simulink model "dyn2"  (R2021b)
settings: Solver=VariableStepAuto  StartTime=0.0  StopTime=10.0  RelTol=1e-3
InitFcn:
  | m=5;
  | I=[0.5 0 0; 0 0.5 0; 0 0 1];
  | c_t=0.02;
  | c_m=0.005;
  | h_i=10;
  | g=9.80665;
  | rho=1;
  | omega_hover=sqrt(m*g/(4*0.5*c_t));
  | a_x=0;
  | a_y=0;
  | a_z=0;
  | a_r=0;
  | a_p=0;
  | a_yaw=0;
  | casee=1;
  | x_i=0;
  | y_i=0;
  | z_i=-10;
  | r_i=0;
  | p_i=90;
  | yaw_i=0;
  | x_f=1;
  | y_f=0;
  | z_f=-10;
  | r_f=0;
  | p_f=90;
  | yaw_f=0;
undefined symbols (not defined in the file or in its folder): X, Y, Z
libraries: sm_lib x32, nesl_utility x11, slpidlib x6
(part 1 of 2)
settings Model: Creator=zafar  LastModifiedBy=zafar

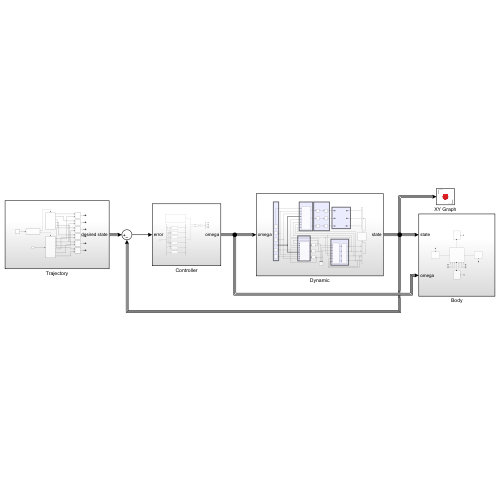
[thumbnail: Simulink's stored preview of the top-level diagram]
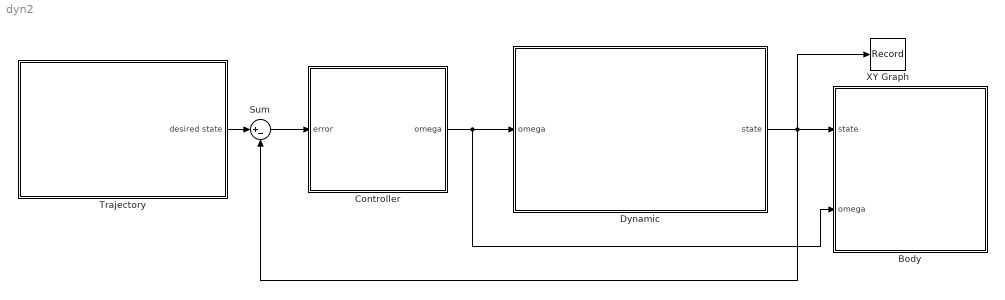
== system dyn2 ==
  Body : Subsystem
  Controller : Subsystem
  Dynamic : Subsystem
  Sum : Sum  Inputs=|+-
  Trajectory : Subsystem
  XY Graph : Record  FileSettingsInternal="{\"entries\":[{\"content\":{\"excelSettings\":{\"content\":{},\"type\":\"Streamout.ExcelSettings\"}},\"type\":\"Streamout.FileSettingStorage\",\"uuid\":\"d4792fb1-0a1f-4ec5-b838-d1a9abcf2949\"}],\"packageUris\":[\"http://schema.mathworks.com/mf0/streamout_blocks/R2020a\"],\"version\":\"1.0\"}"  Layout=[1 2]  SignalsInternal="{\"entries\":[{\"content\":{\"signals\":[{\"content\":{\"blockPath\":[\"dyn2/XY Graph\"],\"channel\":[],\"dimensions\":[1],\"domain\":\"dyn2/XY Graph\",\"hasChildren\":true,\"lineColor\":\"#139fff\",\"plots\":[],\"port\":1,\"sid\":[\"\"],\"signalID\":683,\"signalName\":\"Dynamic\"},\"type\":\"RecordBlkView.Signal\",\"uuid\":\"e1957810-dc31-4c74-8302-1d5d707b7b59\"},{\"content\":{\"blockPath\":[\"dyn2/XY Graph\"],\"channel\":[],\"dimensions\":[1],\"domain\":\"dyn2/XY Graph\",\"leafPath\":\"Dynamic.roll\",\"lineColor\":\"#ff6929\",\"parentID\":683,\"plots\":[9],\"port\":1,\"sid\":[\"\"],\"signalID\":689,\"signalName\":\"Dynamic.roll\"},\"type\":\"RecordBlkView.Signal\",\"uuid\":\"85618280-ea2e-4b5a-aaad-2ba74497e0b1\"},{\"content\":{\"blockPath\":[\"dyn2/XY Graph\"],\"channel\":[],\"dimensions\":[1],\"domain\":\"dyn2/XY Graph\",\"leafPath\":\"Dynamic.pitch\",\"lineColor\":\"#b746ff\",\"parentID\":683,\"plots\":[9],\"port\":1,\"sid\":[\"\"],\"signalID\":693,\"signalName\":\"Dynamic.pitch\"},\"type\":\"RecordBlkView.Signal\",\"uuid\":\"18941b2a-ec3b-4b33-bc23-00b06118022f\"},{\"content\":{\"blockPath\":[\"dyn2/XY Graph\"],\"channel\":[],\"dimensions\":[1],\"domain\":\"dyn2/XY Graph\",\"leafPath\":\"Dynamic.yaw\",\"lineColor\":\"#64d413\",\"parentID\":683,\"plots\":[9],\"port\":1,\"sid\":[\"\"],\"signalID\":697,\"signalName\":\"Dynamic.yaw\"},\"type\":\"RecordBlkView.Signal\",\"uuid\":\"7d2db7da-f018-4d39-9722-8c8cb8260ba4\"},{\"content\":{\"blockPath\":[\"dyn2/XY Graph\"],\"channel\":[],\"dimensions\":[1],\"domain\":\"dyn2/XY Graph\",\"leafPath\":\"Dynamic.x\",\"lineColor\":\"#ff13a6\",\"parentID\":683,\"plots\":[1],\"port\":1,\"sid\":[\"\"],\"signalID\":701,\"signalName\":\"Dynamic.x\"},\"type\":\"RecordBlkView.Signal\",\"uuid\":\"06cf0755-9d67-498c-9d15-2dd6aaf754d1\"},{\"content\":{\"blockPath\":[\"dyn2/XY Graph\"],\"channel\":[],\"dimensions\":[1],\"domain\":\"dyn2/XY Graph\",\"leafPath\":\"Dynamic.y\",\"lineColor\":\"#fe330a\",\"parentID\":683,\"plots\":[1],\"port\":1,\"sid\":[\"\"],\"signalID\":705,\"signalName\":\"Dynamic.y\"},\"type\":\"RecordBlkView.Signal\",\"uuid\":\"010e3232-da4b-4a82-8d08-832df45afe02\"},{\"content\":{\"blockPath\":[\"dyn2/XY Graph\"],\"channel\":[],\"dimensions\":[1],\"domain\":\"dyn2/XY Graph\",\"leafPath\":\"Dynamic.z\",\"lineColor\":\"#22b573\",\"parentID\":683,\"plots\":[1],\"port\":1,\"sid\":[\"\"],\"signalID\":709,\"signalName\":\"Dynamic.z\"},\"type\":\"RecordBlkView.Signal\",\"uuid\":\"f4e3abf7-5929-44e1-b69c-6cdf4737284f\"}]},\"type\":\"RecordBlkView.InputSignals\",\"uuid\":\"78fd29e7-ed61-4860-890e-9c6bc17d912c\"}],\"packageUris\":[\"http://schema.mathworks.com/mf0/streamout_blocks/R2020a\"],\"version\":\"1.0\"}"  CompatibilityTag=XY
  wires:
  Dynamic/1(state) -> XY Graph/1, Sum/2, Body/1(state)
  Controller/1(omega) -> Body/2(omega), Dynamic/1(omega)
  Trajectory/1(desired state) -> Sum/1
  Sum/1 -> Controller/1(error)

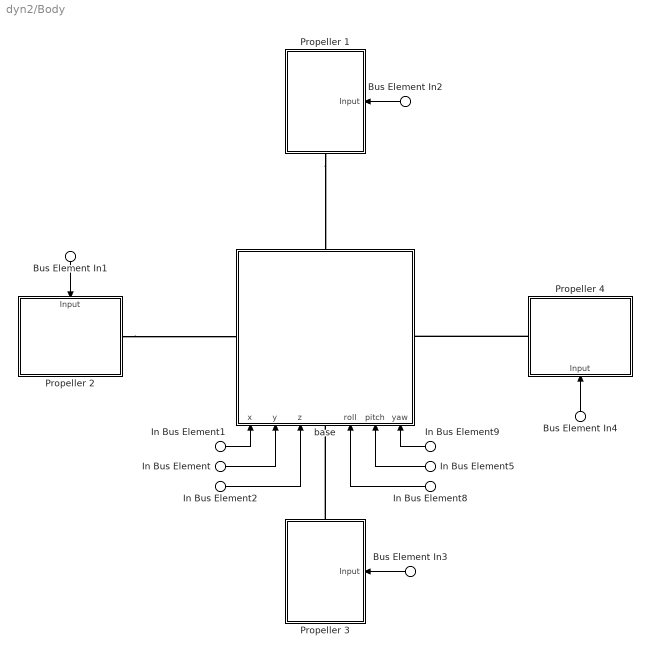
== system dyn2/Body ==
  In Bus Element2 : Inport  PortName=state  Element=z
  In Bus Element1 : Inport  PortName=state  Element=x
  In Bus Element9 : Inport  PortName=state  Element=yaw
  In Bus Element8 : Inport  PortName=state  Element=roll
  In Bus Element5 : Inport  PortName=state  Element=pitch
  In Bus Element : Inport  PortName=state  Element=y
  Bus Element In2 : Inport  Port=2  PortName=omega  Element=omega1
  Bus Element In1 : Inport  Port=2  PortName=omega  Element=omega2
  Bus Element In3 : Inport  Port=2  PortName=omega  Element=omega3
  Bus Element In4 : Inport  Port=2  PortName=omega  Element=omega4
  Propeller 1 : Subsystem
      settings: PortSchema="{\"entries\":[{\"content\":{\"sides\":[{\"content\":{\"connectorIds\":[\"LConn1\"]},\"type\":\"ConnectorPlacement.EquallySpacedRectSide\",\"uuid\":\"cdf25c99-c2c9-48d7-87ea-f6e3a99d1ccc\"},{\"content\":{\"connectorIds\":[],\"side\":\"RIGHT\"},\"type\":\"ConnectorPlacement.EquallySpacedRectSide\",\"uuid\":\"40e1c002-c04a-4a5a-8e9c-b357988226a7\"},{\"content\":{\"connectorIds\":[],\"side\":\"TOP\"},\"type\":\"ConnectorPlacement.EquallySpacedRectSide\",\"uuid\":\"eab61d94-1bf1-42a1-b49f-e701cda87405\"},{\"content\":{\"connectorIds\":[\"In1\"],\"side\":\"BOTTOM\"},\"type\":\"ConnectorPlacement.EquallySpacedRectSide\",\"uuid\":\"d4baf7fe-500e-43b3-b49d-f7ceb4534939\"}]},\"type\":\"ConnectorPlacement.EquallySpacedConnector\",\"uuid\":\"1942d34c-f553-4d78-8efb-5354772d0834\"}],\"packageUris\":[\"http://schema.mathworks.com/mf0/Connector/R2020b\"],\"version\":\"1.0\"}"
  Propeller 2 : Subsystem
      settings: PortSchema="{\"entries\":[{\"content\":{\"sides\":[{\"content\":{\"connectorIds\":[\"LConn1\"]},\"type\":\"ConnectorPlacement.EquallySpacedRectSide\",\"uuid\":\"cdf25c99-c2c9-48d7-87ea-f6e3a99d1ccc\"},{\"content\":{\"connectorIds\":[],\"side\":\"RIGHT\"},\"type\":\"ConnectorPlacement.EquallySpacedRectSide\",\"uuid\":\"40e1c002-c04a-4a5a-8e9c-b357988226a7\"},{\"content\":{\"connectorIds\":[\"In1\"],\"side\":\"TOP\"},\"type\":\"ConnectorPlacement.EquallySpacedRectSide\",\"uuid\":\"eab61d94-1bf1-42a1-b49f-e701cda87405\"}]},\"type\":\"ConnectorPlacement.EquallySpacedConnector\",\"uuid\":\"1942d34c-f553-4d78-8efb-5354772d0834\"}],\"packageUris\":[\"http://schema.mathworks.com/mf0/Connector/R2020b\"],\"version\":\"1.0\"}"
  Propeller 3 : Subsystem
      settings: PortSchema="{\"entries\":[{\"content\":{\"sides\":[{\"content\":{\"connectorIds\":[\"LConn1\"]},\"type\":\"ConnectorPlacement.EquallySpacedRectSide\",\"uuid\":\"cdf25c99-c2c9-48d7-87ea-f6e3a99d1ccc\"},{\"content\":{\"connectorIds\":[],\"side\":\"RIGHT\"},\"type\":\"ConnectorPlacement.EquallySpacedRectSide\",\"uuid\":\"40e1c002-c04a-4a5a-8e9c-b357988226a7\"},{\"content\":{\"connectorIds\":[],\"side\":\"TOP\"},\"type\":\"ConnectorPlacement.EquallySpacedRectSide\",\"uuid\":\"eab61d94-1bf1-42a1-b49f-e701cda87405\"},{\"content\":{\"connectorIds\":[\"In1\"],\"side\":\"BOTTOM\"},\"type\":\"ConnectorPlacement.EquallySpacedRectSide\",\"uuid\":\"d7470312-54f3-4d3a-8a81-0efcc21151e7\"}]},\"type\":\"ConnectorPlacement.EquallySpacedConnector\",\"uuid\":\"1942d34c-f553-4d78-8efb-5354772d0834\"}],\"packageUris\":[\"http://schema.mathworks.com/mf0/Connector/R2020b\"],\"version\":\"1.0\"}"
  Propeller 4 : Subsystem
      settings: PortSchema="{\"entries\":[{\"content\":{\"sides\":[{\"content\":{\"connectorIds\":[\"LConn1\"]},\"type\":\"ConnectorPlacement.EquallySpacedRectSide\",\"uuid\":\"cdf25c99-c2c9-48d7-87ea-f6e3a99d1ccc\"},{\"content\":{\"connectorIds\":[],\"side\":\"RIGHT\"},\"type\":\"ConnectorPlacement.EquallySpacedRectSide\",\"uuid\":\"40e1c002-c04a-4a5a-8e9c-b357988226a7\"},{\"content\":{\"connectorIds\":[],\"side\":\"TOP\"},\"type\":\"ConnectorPlacement.EquallySpacedRectSide\",\"uuid\":\"eab61d94-1bf1-42a1-b49f-e701cda87405\"},{\"content\":{\"connectorIds\":[\"In1\"],\"side\":\"BOTTOM\"},\"type\":\"ConnectorPlacement.EquallySpacedRectSide\",\"uuid\":\"25618f8e-b249-4005-b2d0-d585f13f3048\"}]},\"type\":\"ConnectorPlacement.EquallySpacedConnector\",\"uuid\":\"1942d34c-f553-4d78-8efb-5354772d0834\"}],\"packageUris\":[\"http://schema.mathworks.com/mf0/Connector/R2020b\"],\"version\":\"1.0\"}"
  base : Subsystem
      settings: PortSchema="{\"entries\":[{\"content\":{\"sides\":[{\"content\":{\"connectorIds\":[\"In1\",\"In2\",\"In3\",\"LConn1\",\"In4\",\"In5\",\"In6\"]},\"type\":\"ConnectorPlacement.EquallySpacedRectSide\",\"uuid\":\"779db686-b372-48f2-8e56-3039c1dfa828\"},{\"content\":{\"connectorIds\":[\"RConn1\"],\"side\":\"RIGHT\"},\"type\":\"ConnectorPlacement.EquallySpacedRectSide\",\"uuid\":\"5342d4b0-d4cc-41da-a1a0-0c3712086a6a\"},{\"content\":{\"connectorIds\":[\"LConn2\"],\"side\":\"TOP\"},\"type\":\"ConnectorPlacement.EquallySpacedRectSide\",\"uuid\":\"806fe2cc-07c0-46bb-9d80-26a95cc2c32b\"},{\"content\":{\"connectorIds\":[\"RConn2\"],\"side\":\"BOTTOM\"},\"type\":\"ConnectorPlacement.EquallySpacedRectSide\",\"uuid\":\"aa12e65d-c8a8-4fde-8e0f-187926b8e052\"}]},\"type\":\"ConnectorPlacement.EquallySpacedConnector\",\"uuid\":\"4d2b6a53-689c-48c9-b350-3dab09cbcb7b\"}],\"packageUris\":[\"http://schema.mathworks.com/mf0/Connector/R2020b\"],\"version\":\"1.0\"}"
  wires:
  In Bus Element1/1 -> base/1(x)
  In Bus Element/1 -> base/2(y)
  In Bus Element2/1 -> base/3(z)
  In Bus Element8/1 -> base/4(roll)
  In Bus Element5/1 -> base/5(pitch)
  In Bus Element9/1 -> base/6(yaw)
  Bus Element In2/1 -> Propeller 1/1(Input)
  Bus Element In1/1 -> Propeller 2/1(Input)
  Bus Element In3/1 -> Propeller 3/1(Input)
  Bus Element In4/1 -> Propeller 4/1(Input)
  connections:
  Propeller 4/LConn1 -- base/RConn2
  Propeller 1/LConn1 -- base/RConn1
  Propeller 2/LConn1 -- base/LConn2
  Propeller 3/LConn1 -- base/LConn1

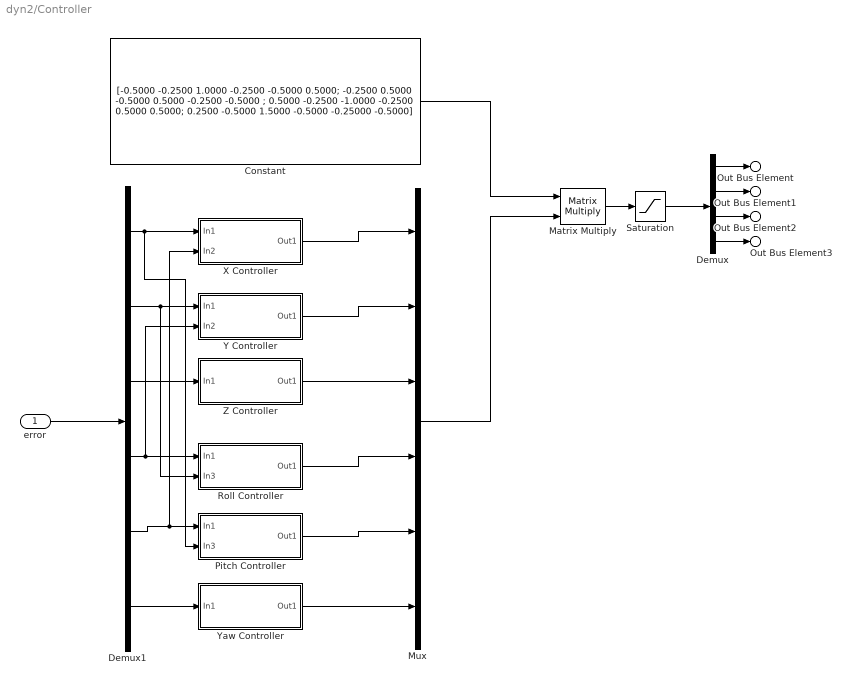
== system dyn2/Controller ==
  error : Inport
  Constant : Constant  Value=|
      | [-0.5000   -0.2500    1.0000   -0.2500   -0.5000    0.5000;
      |    -0.2500    0.5000   -0.5000    0.5000   -0.2500   -0.5000
      | ;    0.5000   -0.2500   -1.0000   -0.2500    0.5000    0.5000;
      |     0.2500   -0.5000    1.5000   -0.5000   -0.25000   -0.5000]
  Demux : Demux
  Demux1 : Demux  Outputs=6
  Matrix Multiply : Product  Multiplication=Matrix(*)
  Mux : Mux  Inputs=6
  Pitch Controller : Subsystem
  Roll Controller : Subsystem
  Saturation : Saturate  UpperLimit=10000  LowerLimit=0
  X Controller : Subsystem
  Y Controller : Subsystem
  Yaw Controller : Subsystem
  Z Controller : Subsystem
  Out Bus Element : Outport  PortName=omega  Element=omega1
  Out Bus Element1 : Outport  PortName=omega  Element=omega2
  Out Bus Element2 : Outport  PortName=omega  Element=omega3
  Out Bus Element3 : Outport  PortName=omega  Element=omega4
  wires:
  Yaw Controller/1(Out1) -> Mux/6
  Pitch Controller/1(Out1) -> Mux/5
  Roll Controller/1(Out1) -> Mux/4
  Z Controller/1(Out1) -> Mux/3
  X Controller/1(Out1) -> Mux/1
  Constant/1 -> Matrix Multiply/1
  Mux/1 -> Matrix Multiply/2
  Matrix Multiply/1 -> Saturation/1
  Saturation/1 -> Demux/1
  Demux/1 -> Out Bus Element/1
  Demux/2 -> Out Bus Element1/1
  Demux/3 -> Out Bus Element2/1
  Demux/4 -> Out Bus Element3/1
  Demux1/1 -> Pitch Controller/2(In3), X Controller/1(In1)
  Demux1/3 -> Z Controller/1(In1)
  Demux1/4 -> Y Controller/2(In2), Roll Controller/1(In1)
  Demux1/5 -> X Controller/2(In2), Pitch Controller/1(In1)
  Demux1/6 -> Yaw Controller/1(In1)
  error/1 -> Demux1/1
  Demux1/2 -> Roll Controller/2(In3), Y Controller/1(In1)
  Y Controller/1(Out1) -> Mux/2

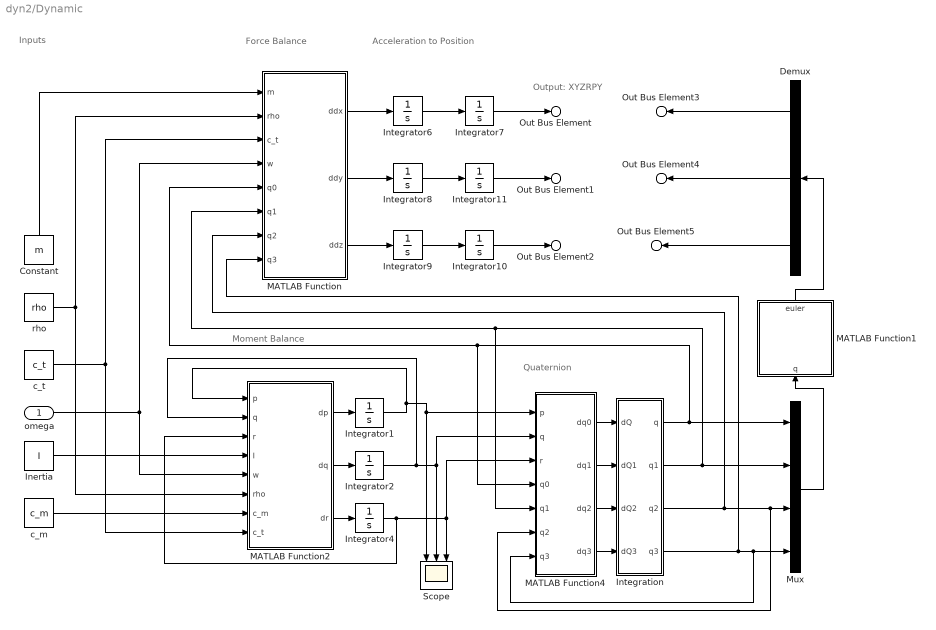
== system dyn2/Dynamic ==
  note: Inputs
  note: Moment Balance
  note: Quaternion
  note: Acceleration to Position
  note: Force Balance
  note: Output: XYZRPY
  omega : Inport
  Constant : Constant  Value=m
  Demux : Demux  Outputs=3
  Inertia : Constant  Value=I
  Integration : Subsystem
  Integrator{1..2,4,6..9,11} (8 alike) : Integrator
  Integrator10 : Integrator  InitialCondition=-h_i
  MATLAB Function : MATLAB Function  TreatAsAtomicUnit=on
  MATLAB Function1 : MATLAB Function  TreatAsAtomicUnit=on
  MATLAB Function2 : MATLAB Function  TreatAsAtomicUnit=on
  MATLAB Function4 : MATLAB Function  TreatAsAtomicUnit=on
  Mux : Mux
  Scope : Scope  NumInputPorts=3
  c_m : Constant  Value=c_m
  c_t : Constant  Value=c_t
  rho : Constant  Value=rho
  Out Bus Element3 : Outport  PortName=state  Element=roll
  Out Bus Element4 : Outport  PortName=state  Element=pitch
  Out Bus Element5 : Outport  PortName=state  Element=yaw
  Out Bus Element : Outport  PortName=state  Element=x
  Out Bus Element1 : Outport  PortName=state  Element=y
  Out Bus Element2 : Outport  PortName=state  Element=z
  wires:
  Mux/1 -> MATLAB Function1/1(q)
  Integration/4(q3) -> Mux/4, MATLAB Function4/7(q3), MATLAB Function/8(q3)
  Integration/3(q2) -> Mux/3, MATLAB Function4/6(q2), MATLAB Function/7(q2)
  Integration/2(q1) -> Mux/2, MATLAB Function4/5(q1), MATLAB Function/6(q1)
  MATLAB Function4/4(dq3) -> Integration/4(dQ3)
  MATLAB Function4/3(dq2) -> Integration/3(dQ2)
  MATLAB Function4/2(dq1) -> Integration/2(dQ1)
  MATLAB Function4/1(dq0) -> Integration/1(dQ)
  Demux/2 -> Out Bus Element4/1
  Demux/3 -> Out Bus Element5/1
  Integrator4/1 -> MATLAB Function4/3(r), Scope/3, MATLAB Function2/3(r)
  MATLAB Function1/1(euler) -> Demux/1
  MATLAB Function/2(ddy) -> Integrator8/1
  Demux/1 -> Out Bus Element3/1
  Constant/1 -> MATLAB Function/1(m)
  rho/1 -> MATLAB Function2/6(rho), MATLAB Function/2(rho)
  c_m/1 -> MATLAB Function2/7(c_m)
  MATLAB Function/3(ddz) -> Integrator9/1
  Integrator1/1 -> MATLAB Function4/1(p), Scope/1, MATLAB Function2/1(p)
  Integration/1(q) -> Mux/1, MATLAB Function4/4(q0), MATLAB Function/5(q0)
  MATLAB Function2/1(dp) -> Integrator1/1
  Integrator10/1 -> Out Bus Element2/1
  MATLAB Function/1(ddx) -> Integrator6/1
  Integrator8/1 -> Integrator11/1
  MATLAB Function2/2(dq) -> Integrator2/1
  Integrator6/1 -> Integrator7/1
  Integrator11/1 -> Out Bus Element1/1
  Integrator7/1 -> Out Bus Element/1
  Integrator2/1 -> MATLAB Function2/2(q), Scope/2, MATLAB Function4/2(q)
  c_t/1 -> MATLAB Function2/8(c_t), MATLAB Function/3(c_t)
  Integrator9/1 -> Integrator10/1
  omega/1 -> MATLAB Function/4(w), MATLAB Function2/5(w)
  MATLAB Function2/3(dr) -> Integrator4/1
  Inertia/1 -> MATLAB Function2/4(I)

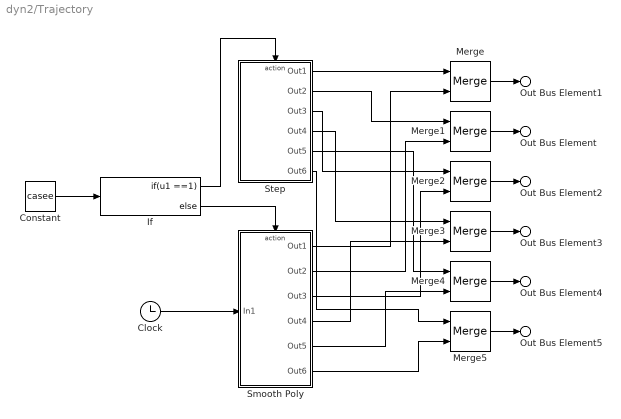
== system dyn2/Trajectory ==
  Clock : Clock
  Constant : Constant  Value=casee
  If : If  IfExpression=u1 ==1
  Merge{,1..5} (6 alike) : Merge
  Smooth Poly : Subsystem  TreatAsAtomicUnit=on
  Step : Subsystem  TreatAsAtomicUnit=on
  Out Bus Element1 : Outport  PortName=desired state  Element=x
  Out Bus Element : Outport  PortName=desired state  Element=y
  Out Bus Element2 : Outport  PortName=desired state  Element=z
  Out Bus Element3 : Outport  PortName=desired state  Element=roll
  Out Bus Element4 : Outport  PortName=desired state  Element=pitch
  Out Bus Element5 : Outport  PortName=desired state  Element=yaw
  wires:
  Smooth Poly/3(Out3) -> Merge2/2
  Step/3(Out3) -> Merge2/1
  Smooth Poly/2(Out2) -> Merge1/2
  Step/2(Out2) -> Merge1/1
  Smooth Poly/1(Out1) -> Merge/2
  Step/1(Out1) -> Merge/1
  If/2 -> Smooth Poly/Action
  If/1 -> Step/Action
  Constant/1 -> If/1
  Clock/1 -> Smooth Poly/1(In1)
  Step/4(Out4) -> Merge3/1
  Smooth Poly/4(Out4) -> Merge3/2
  Smooth Poly/5(Out5) -> Merge4/2
  Step/5(Out5) -> Merge4/1
  Step/6(Out6) -> Merge5/1
  Smooth Poly/6(Out6) -> Merge5/2
  Merge/1 -> Out Bus Element1/1
  Merge1/1 -> Out Bus Element/1
  Merge2/1 -> Out Bus Element2/1
  Merge3/1 -> Out Bus Element3/1
  Merge4/1 -> Out Bus Element4/1
  Merge5/1 -> Out Bus Element5/1

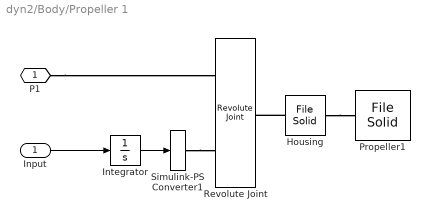
== system dyn2/Body/Propeller 1 ==
  Input : Inport
  Housing : sm_lib/Body Elements/File Solid  ExtGeomFileName=E:\tosort\aerial\my new version\motor.STEP  UnitType=FromFile  ExtGeomFileUnits=m  StepReaderType=HEX  ExportConvexHullGeometry=off  InertiaType=Custom  Mass=51  MassUnits=g  CenterOfMass=[0, 0, -0.0088876]  CenterOfMassUnits=m  MomentsOfInertia=[7.0438e-06, 7.04379e-06, 6.06908e-06]  MomentsOfInertiaUnits=kg*m^2  ProductsOfInertia=[0 0 0]  ProductsOfInertiaUnits=kg*m^2  BasedOnType=Mass  Density=1000  DensityUnits=kg/m^3  DoExposeReferenceFrame=off  SerializedFrames=<Frames><Frame><Id>Frame1</Id><Value><Name>F1</Name><Origin><Source>GeometricFeature</Source><FeatureName>planar surface 3</FeatureName></Origin><PrimaryAxis><DefinedDirection>+Z</DefinedDirection><Source>ReferenceFrame</Source><SourceDirection>+Z</SourceDirection><FeatureName></FeatureName></PrimaryAxis><SecondaryAxis><DefinedDirection>+X</DefinedDirection><Source>ReferenceFrame</Source><SourceDirection>+X</SourceDirection><FeatureName></FeatureName></SecondaryAxis></Value></Frame><Frame><Id>Frame2</Id><Value><Name>F2</Name><Origin><Source>GeometricFeature</Source><FeatureName>circular curve 1</FeatureName></Origin><PrimaryAxis><DefinedDirection>+Z</DefinedDirection><Source>ReferenceFrame</Source><SourceDirection>+Z</SourceDirection><FeatureName></FeatureName></PrimaryAxis><SecondaryAxis><DefinedDirection>+X</DefinedDirection><Source>ReferenceFrame</Source><SourceDirection>+X</SourceDirection><FeatureName></FeatureName></SecondaryAxis></Value></Frame></Frames>  GraphicType=FromGeometry  MarkerShape=Sphere  MarkerSize=10  GraphicVisPropType=SimpleVisualProperties  GraphicDiffuseColor=[0.6 0.0 0.2]  GraphicSpecularColor=[0.5 0.5 0.5 1.0]  GraphicAmbientColor=[0.15 0.15 0.15 1.0]  GraphicEmissiveColor=[0.0 0.0 0.0 1.0]  GraphicShininess=75  GraphicOpacity=1.0
  Integrator : Integrator
  Propeller1 : sm_lib/Body Elements/File Solid  ExtGeomFileName=E:\tosort\aerial\my new version\propeller.STEP  UnitType=FromFile  ExtGeomFileUnits=m  StepReaderType=HEX  ExportConvexHullGeometry=off  InertiaType=Custom  Mass=0.0249468  MassUnits=kg  CenterOfMass="[0  0.00566766 0]"  CenterOfMassUnits=m  MomentsOfInertia=[0.000160013, 0.000160582, 8.20018e-07]  MomentsOfInertiaUnits=kg*m^2  ProductsOfInertia=[0 0 0]  ProductsOfInertiaUnits=kg*m^2  BasedOnType=Density  Density=1  DensityUnits=g/cm^3  DoExposeReferenceFrame=off  SerializedFrames=<Frames><Frame><Id>Frame1</Id><Value><Name>F1</Name><Origin><Source>GeometricFeature</Source><FeatureName>circular curve 14</FeatureName></Origin><PrimaryAxis><DefinedDirection>+Z</DefinedDirection><Source>ReferenceFrame</Source><SourceDirection>+Y</SourceDirection><FeatureName></FeatureName></PrimaryAxis><SecondaryAxis><DefinedDirection>+X</DefinedDirection><Source>ReferenceFrame</Source><SourceDirection>+X</SourceDirection><FeatureName></FeatureName></SecondaryAxis></Value></Frame></Frames>  GraphicType=FromGeometry  MarkerShape=Sphere  MarkerSize=10  GraphicVisPropType=AdvancedVisualProperties  GraphicDiffuseColor=[0.05 0.05 0.05]  GraphicSpecularColor=[0.5 0.5 0.5 1.0]  GraphicAmbientColor=[0.15 0.15 0.15 1.0]  GraphicEmissiveColor=[0.0 0.0 0.0 1.0]  GraphicShininess=40  GraphicOpacity=1.0
  Revolute Joint : sm_lib/Joints/Revolute Joint  JointMode=Normal  SenseConstraintForce=off  SenseConstraintForceX=off  SenseConstraintForceY=off  SenseConstraintForceZ=off  SenseConstraintTorque=off  SenseConstraintTorqueX=off  SenseConstraintTorqueY=off  SenseConstraintTorqueZ=off  SenseTotalForce=off  SenseTotalForceX=off  SenseTotalForceY=off  SenseTotalForceZ=off  SenseTotalTorque=off  SenseTotalTorqueX=off  SenseTotalTorqueY=off  SenseTotalTorqueZ=off  CompositeWrenchDir=FollowerOnBase  CompositeWrenchFrame=BaseFrame  EquilibriumPosition=0  EquilibriumPositionUnits=deg  SpringStiffness=0  SpringStiffnessUnits=N*m/rad  DampingCoefficient=1e-5  DampingCoefficientUnits=N*m/(rad/s)  TorqueActuationMode=ComputedTorque  MotionActuationMode=InputMotion  SensePosition=off  SenseVelocity=off  SenseAcceleration=off  SenseTorqueForce=off  SenseLowerLimitTorqueForce=off  SenseUpperLimitTorqueForce=off  LowerLimitSpecify=off  LowerLimitBound=-90  LowerLimitBoundUnits=deg  LowerLimitStiffness=1e4  LowerLimitStiffnessUnits=N*m/deg  LowerLimitDamping=10  LowerLimitDampingUnits=N*m/(deg/s)  LowerLimitTransitionRegionWidth=0.1  LowerLimitTransitionRegionWidthUnits=deg  UpperLimitSpecify=off  UpperLimitBound=90  UpperLimitBoundUnits=deg  UpperLimitStiffness=1e4  UpperLimitStiffnessUnits=N*m/deg  UpperLimitDamping=10  UpperLimitDampingUnits=N*m/(deg/s)  UpperLimitTransitionRegionWidth=0.1  UpperLimitTransitionRegionWidthUnits=deg  PositionTargetSpecify=off  PositionTargetPriority=High  PositionTargetValue=0  PositionTargetValueUnits=deg  VelocityTargetSpecify=off  VelocityTargetPriority=High  VelocityTargetValue=0  VelocityTargetValueUnits=deg/s
  Simulink-PS Converter1 : nesl_utility/Simulink-PS Converter  PhysicalDomain=network_engine_domain  SubClassName=ps_input  LeftPortType=input  RightPortType=output  PseudoPeriodic=off  Frequencies=[]  NoiseDistribution=none  NoiseParameters=[]  Unit=rad  AffineConversion=off  FilteringAndDerivatives=filter  SimscapeFilterOrder=2  InputFilterTimeConstant=0.001  UdotUserProvided=0
      settings: SourceProductBaseCode=PW,SS
  P1 : PMIOPort  Side=Left
  wires:
  Input/1 -> Integrator/1
  Integrator/1 -> Simulink-PS Converter1/1
  connections:
  Housing/RConn1 -- Propeller1/LConn1
  P1/RConn1 -- Revolute Joint/LConn1
  Housing/LConn1 -- Revolute Joint/RConn1
  Simulink-PS Converter1/RConn1 -- Revolute Joint/LConn2

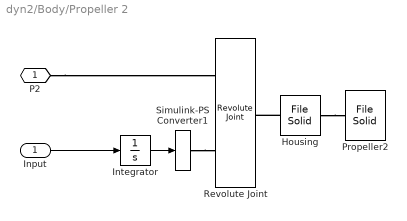
== system dyn2/Body/Propeller 2 ==
  Input : Inport
  Housing : sm_lib/Body Elements/File Solid  ExtGeomFileName=E:\tosort\aerial\my new version\motor.STEP  UnitType=FromFile  ExtGeomFileUnits=m  StepReaderType=HEX  ExportConvexHullGeometry=off  InertiaType=Custom  Mass=51  MassUnits=g  CenterOfMass=[0, 0, -0.0088876]  CenterOfMassUnits=m  MomentsOfInertia=[7.0438e-06, 7.04379e-06, 6.06908e-06]  MomentsOfInertiaUnits=kg*m^2  ProductsOfInertia=[0 0 0]  ProductsOfInertiaUnits=kg*m^2  BasedOnType=Mass  Density=1000  DensityUnits=kg/m^3  DoExposeReferenceFrame=off  SerializedFrames=<Frames><Frame><Id>Frame1</Id><Value><Name>F1</Name><Origin><Source>GeometricFeature</Source><FeatureName>planar surface 3</FeatureName></Origin><PrimaryAxis><DefinedDirection>+Z</DefinedDirection><Source>ReferenceFrame</Source><SourceDirection>+Z</SourceDirection><FeatureName></FeatureName></PrimaryAxis><SecondaryAxis><DefinedDirection>+X</DefinedDirection><Source>ReferenceFrame</Source><SourceDirection>+X</SourceDirection><FeatureName></FeatureName></SecondaryAxis></Value></Frame><Frame><Id>Frame2</Id><Value><Name>F2</Name><Origin><Source>GeometricFeature</Source><FeatureName>circular curve 1</FeatureName></Origin><PrimaryAxis><DefinedDirection>+Z</DefinedDirection><Source>ReferenceFrame</Source><SourceDirection>+Z</SourceDirection><FeatureName></FeatureName></PrimaryAxis><SecondaryAxis><DefinedDirection>+X</DefinedDirection><Source>ReferenceFrame</Source><SourceDirection>+X</SourceDirection><FeatureName></FeatureName></SecondaryAxis></Value></Frame></Frames>  GraphicType=FromGeometry  MarkerShape=Sphere  MarkerSize=10  GraphicVisPropType=SimpleVisualProperties  GraphicDiffuseColor=[0.6 0.0 0.2]  GraphicSpecularColor=[0.5 0.5 0.5 1.0]  GraphicAmbientColor=[0.15 0.15 0.15 1.0]  GraphicEmissiveColor=[0.0 0.0 0.0 1.0]  GraphicShininess=75  GraphicOpacity=1.0
  Integrator : Integrator
  Propeller2 : sm_lib/Body Elements/File Solid  ExtGeomFileName=E:\tosort\aerial\my new version\propeller.STEP  UnitType=FromFile  ExtGeomFileUnits=m  StepReaderType=HEX  ExportConvexHullGeometry=off  InertiaType=Custom  Mass=0.0249468  MassUnits=kg  CenterOfMass="[0  0.00566766 0]"  CenterOfMassUnits=m  MomentsOfInertia=[0.000160013, 0.000160582, 8.20018e-07]  MomentsOfInertiaUnits=kg*m^2  ProductsOfInertia=[0 0 0]  ProductsOfInertiaUnits=kg*m^2  BasedOnType=Density  Density=1  DensityUnits=g/cm^3  DoExposeReferenceFrame=off  SerializedFrames=<Frames><Frame><Id>Frame1</Id><Value><Name>F1</Name><Origin><Source>GeometricFeature</Source><FeatureName>circular curve 14</FeatureName></Origin><PrimaryAxis><DefinedDirection>+Z</DefinedDirection><Source>ReferenceFrame</Source><SourceDirection>+Y</SourceDirection><FeatureName></FeatureName></PrimaryAxis><SecondaryAxis><DefinedDirection>+X</DefinedDirection><Source>ReferenceFrame</Source><SourceDirection>+X</SourceDirection><FeatureName></FeatureName></SecondaryAxis></Value></Frame></Frames>  GraphicType=FromGeometry  MarkerShape=Sphere  MarkerSize=10  GraphicVisPropType=AdvancedVisualProperties  GraphicDiffuseColor=[0.05 0.05 0.05]  GraphicSpecularColor=[0.5 0.5 0.5 1.0]  GraphicAmbientColor=[0.15 0.15 0.15 1.0]  GraphicEmissiveColor=[0.0 0.0 0.0 1.0]  GraphicShininess=40  GraphicOpacity=1.0
  Revolute Joint : sm_lib/Joints/Revolute Joint  JointMode=Normal  SenseConstraintForce=off  SenseConstraintForceX=off  SenseConstraintForceY=off  SenseConstraintForceZ=off  SenseConstraintTorque=off  SenseConstraintTorqueX=off  SenseConstraintTorqueY=off  SenseConstraintTorqueZ=off  SenseTotalForce=off  SenseTotalForceX=off  SenseTotalForceY=off  SenseTotalForceZ=off  SenseTotalTorque=off  SenseTotalTorqueX=off  SenseTotalTorqueY=off  SenseTotalTorqueZ=off  CompositeWrenchDir=FollowerOnBase  CompositeWrenchFrame=BaseFrame  EquilibriumPosition=0  EquilibriumPositionUnits=deg  SpringStiffness=0  SpringStiffnessUnits=N*m/rad  DampingCoefficient=1e-5  DampingCoefficientUnits=N*m/(rad/s)  TorqueActuationMode=ComputedTorque  MotionActuationMode=InputMotion  SensePosition=off  SenseVelocity=off  SenseAcceleration=off  SenseTorqueForce=off  SenseLowerLimitTorqueForce=off  SenseUpperLimitTorqueForce=off  LowerLimitSpecify=off  LowerLimitBound=-90  LowerLimitBoundUnits=deg  LowerLimitStiffness=1e4  LowerLimitStiffnessUnits=N*m/deg  LowerLimitDamping=10  LowerLimitDampingUnits=N*m/(deg/s)  LowerLimitTransitionRegionWidth=0.1  LowerLimitTransitionRegionWidthUnits=deg  UpperLimitSpecify=off  UpperLimitBound=90  UpperLimitBoundUnits=deg  UpperLimitStiffness=1e4  UpperLimitStiffnessUnits=N*m/deg  UpperLimitDamping=10  UpperLimitDampingUnits=N*m/(deg/s)  UpperLimitTransitionRegionWidth=0.1  UpperLimitTransitionRegionWidthUnits=deg  PositionTargetSpecify=off  PositionTargetPriority=High  PositionTargetValue=0  PositionTargetValueUnits=deg  VelocityTargetSpecify=off  VelocityTargetPriority=High  VelocityTargetValue=0  VelocityTargetValueUnits=deg/s
  Simulink-PS Converter1 : nesl_utility/Simulink-PS Converter  PhysicalDomain=network_engine_domain  SubClassName=ps_input  LeftPortType=input  RightPortType=output  PseudoPeriodic=off  Frequencies=[]  NoiseDistribution=none  NoiseParameters=[]  Unit=rad  AffineConversion=off  FilteringAndDerivatives=filter  SimscapeFilterOrder=2  InputFilterTimeConstant=0.001  UdotUserProvided=0
      settings: SourceProductBaseCode=PW,SS
  P2 : PMIOPort  Side=Left
  wires:
  Integrator/1 -> Simulink-PS Converter1/1
  Input/1 -> Integrator/1
  connections:
  Simulink-PS Converter1/RConn1 -- Revolute Joint/LConn2
  Housing/LConn1 -- Revolute Joint/RConn1
  P2/RConn1 -- Revolute Joint/LConn1
  Housing/RConn1 -- Propeller2/LConn1

== system dyn2/Body/Propeller 3 ==
  Input : Inport
  Housing : sm_lib/Body Elements/File Solid  ExtGeomFileName=E:\tosort\aerial\my new version\motor.STEP  UnitType=FromFile  ExtGeomFileUnits=m  StepReaderType=HEX  ExportConvexHullGeometry=off  InertiaType=Custom  Mass=51  MassUnits=g  CenterOfMass=[0, 0, -0.0088876]  CenterOfMassUnits=m  MomentsOfInertia=[7.0438e-06, 7.04379e-06, 6.06908e-06]  MomentsOfInertiaUnits=kg*m^2  ProductsOfInertia=[0 0 0]  ProductsOfInertiaUnits=kg*m^2  BasedOnType=Mass  Density=1000  DensityUnits=kg/m^3  DoExposeReferenceFrame=off  SerializedFrames=<Frames><Frame><Id>Frame1</Id><Value><Name>F1</Name><Origin><Source>GeometricFeature</Source><FeatureName>planar surface 3</FeatureName></Origin><PrimaryAxis><DefinedDirection>+Z</DefinedDirection><Source>ReferenceFrame</Source><SourceDirection>+Z</SourceDirection><FeatureName></FeatureName></PrimaryAxis><SecondaryAxis><DefinedDirection>+X</DefinedDirection><Source>ReferenceFrame</Source><SourceDirection>+X</SourceDirection><FeatureName></FeatureName></SecondaryAxis></Value></Frame><Frame><Id>Frame2</Id><Value><Name>F2</Name><Origin><Source>GeometricFeature</Source><FeatureName>circular curve 1</FeatureName></Origin><PrimaryAxis><DefinedDirection>+Z</DefinedDirection><Source>ReferenceFrame</Source><SourceDirection>+Z</SourceDirection><FeatureName></FeatureName></PrimaryAxis><SecondaryAxis><DefinedDirection>+X</DefinedDirection><Source>ReferenceFrame</Source><SourceDirection>+X</SourceDirection><FeatureName></FeatureName></SecondaryAxis></Value></Frame></Frames>  GraphicType=FromGeometry  MarkerShape=Sphere  MarkerSize=10  GraphicVisPropType=SimpleVisualProperties  GraphicDiffuseColor=[0.6 0.0 0.2]  GraphicSpecularColor=[0.5 0.5 0.5 1.0]  GraphicAmbientColor=[0.15 0.15 0.15 1.0]  GraphicEmissiveColor=[0.0 0.0 0.0 1.0]  GraphicShininess=75  GraphicOpacity=1.0
  Integrator : Integrator
  Propeller3 : sm_lib/Body Elements/File Solid  ExtGeomFileName=E:\tosort\aerial\my new version\propeller.STEP  UnitType=FromFile  ExtGeomFileUnits=m  StepReaderType=HEX  ExportConvexHullGeometry=off  InertiaType=Custom  Mass=0.0249468  MassUnits=kg  CenterOfMass="[0  0.00566766 0]"  CenterOfMassUnits=m  MomentsOfInertia=[0.000160013, 0.000160582, 8.20018e-07]  MomentsOfInertiaUnits=kg*m^2  ProductsOfInertia=[0 0 0]  ProductsOfInertiaUnits=kg*m^2  BasedOnType=Density  Density=1  DensityUnits=g/cm^3  DoExposeReferenceFrame=off  SerializedFrames=<Frames><Frame><Id>Frame1</Id><Value><Name>F1</Name><Origin><Source>GeometricFeature</Source><FeatureName>circular curve 14</FeatureName></Origin><PrimaryAxis><DefinedDirection>+Z</DefinedDirection><Source>ReferenceFrame</Source><SourceDirection>+Y</SourceDirection><FeatureName></FeatureName></PrimaryAxis><SecondaryAxis><DefinedDirection>+X</DefinedDirection><Source>ReferenceFrame</Source><SourceDirection>+X</SourceDirection><FeatureName></FeatureName></SecondaryAxis></Value></Frame></Frames>  GraphicType=FromGeometry  MarkerShape=Sphere  MarkerSize=10  GraphicVisPropType=AdvancedVisualProperties  GraphicDiffuseColor=[0.05 0.05 0.05]  GraphicSpecularColor=[0.5 0.5 0.5 1.0]  GraphicAmbientColor=[0.15 0.15 0.15 1.0]  GraphicEmissiveColor=[0.0 0.0 0.0 1.0]  GraphicShininess=40  GraphicOpacity=1.0
  Revolute Joint : sm_lib/Joints/Revolute Joint  JointMode=Normal  SenseConstraintForce=off  SenseConstraintForceX=off  SenseConstraintForceY=off  SenseConstraintForceZ=off  SenseConstraintTorque=off  SenseConstraintTorqueX=off  SenseConstraintTorqueY=off  SenseConstraintTorqueZ=off  SenseTotalForce=off  SenseTotalForceX=off  SenseTotalForceY=off  SenseTotalForceZ=off  SenseTotalTorque=off  SenseTotalTorqueX=off  SenseTotalTorqueY=off  SenseTotalTorqueZ=off  CompositeWrenchDir=FollowerOnBase  CompositeWrenchFrame=BaseFrame  EquilibriumPosition=0  EquilibriumPositionUnits=deg  SpringStiffness=0  SpringStiffnessUnits=N*m/rad  DampingCoefficient=1e-5  DampingCoefficientUnits=N*m/(rad/s)  TorqueActuationMode=ComputedTorque  MotionActuationMode=InputMotion  SensePosition=off  SenseVelocity=off  SenseAcceleration=off  SenseTorqueForce=off  SenseLowerLimitTorqueForce=off  SenseUpperLimitTorqueForce=off  LowerLimitSpecify=off  LowerLimitBound=-90  LowerLimitBoundUnits=deg  LowerLimitStiffness=1e4  LowerLimitStiffnessUnits=N*m/deg  LowerLimitDamping=10  LowerLimitDampingUnits=N*m/(deg/s)  LowerLimitTransitionRegionWidth=0.1  LowerLimitTransitionRegionWidthUnits=deg  UpperLimitSpecify=off  UpperLimitBound=90  UpperLimitBoundUnits=deg  UpperLimitStiffness=1e4  UpperLimitStiffnessUnits=N*m/deg  UpperLimitDamping=10  UpperLimitDampingUnits=N*m/(deg/s)  UpperLimitTransitionRegionWidth=0.1  UpperLimitTransitionRegionWidthUnits=deg  PositionTargetSpecify=off  PositionTargetPriority=High  PositionTargetValue=0  PositionTargetValueUnits=deg  VelocityTargetSpecify=off  VelocityTargetPriority=High  VelocityTargetValue=0  VelocityTargetValueUnits=deg/s
  Simulink-PS Converter1 : nesl_utility/Simulink-PS Converter  PhysicalDomain=network_engine_domain  SubClassName=ps_input  LeftPortType=input  RightPortType=output  PseudoPeriodic=off  Frequencies=[]  NoiseDistribution=none  NoiseParameters=[]  Unit=rad  AffineConversion=off  FilteringAndDerivatives=filter  SimscapeFilterOrder=2  InputFilterTimeConstant=0.001  UdotUserProvided=0
      settings: SourceProductBaseCode=PW,SS
  P3 : PMIOPort  Side=Left
  wires:
  Input/1 -> Integrator/1
  Integrator/1 -> Simulink-PS Converter1/1
  connections:
  Housing/RConn1 -- Propeller3/LConn1
  P3/RConn1 -- Revolute Joint/LConn1
  Housing/LConn1 -- Revolute Joint/RConn1
  Simulink-PS Converter1/RConn1 -- Revolute Joint/LConn2

== system dyn2/Body/Propeller 4 ==
  Input : Inport
  Housing : sm_lib/Body Elements/File Solid  ExtGeomFileName=E:\tosort\aerial\my new version\motor.STEP  UnitType=FromFile  ExtGeomFileUnits=m  StepReaderType=HEX  ExportConvexHullGeometry=off  InertiaType=Custom  Mass=51  MassUnits=g  CenterOfMass=[0, 0, -0.0088876]  CenterOfMassUnits=m  MomentsOfInertia=[7.0438e-06, 7.04379e-06, 6.06908e-06]  MomentsOfInertiaUnits=kg*m^2  ProductsOfInertia=[0 0 0]  ProductsOfInertiaUnits=kg*m^2  BasedOnType=Mass  Density=1000  DensityUnits=kg/m^3  DoExposeReferenceFrame=off  SerializedFrames=<Frames><Frame><Id>Frame1</Id><Value><Name>F1</Name><Origin><Source>GeometricFeature</Source><FeatureName>planar surface 3</FeatureName></Origin><PrimaryAxis><DefinedDirection>+Z</DefinedDirection><Source>ReferenceFrame</Source><SourceDirection>+Z</SourceDirection><FeatureName></FeatureName></PrimaryAxis><SecondaryAxis><DefinedDirection>+X</DefinedDirection><Source>ReferenceFrame</Source><SourceDirection>+X</SourceDirection><FeatureName></FeatureName></SecondaryAxis></Value></Frame><Frame><Id>Frame2</Id><Value><Name>F2</Name><Origin><Source>GeometricFeature</Source><FeatureName>circular curve 1</FeatureName></Origin><PrimaryAxis><DefinedDirection>+Z</DefinedDirection><Source>ReferenceFrame</Source><SourceDirection>+Z</SourceDirection><FeatureName></FeatureName></PrimaryAxis><SecondaryAxis><DefinedDirection>+X</DefinedDirection><Source>ReferenceFrame</Source><SourceDirection>+X</SourceDirection><FeatureName></FeatureName></SecondaryAxis></Value></Frame></Frames>  GraphicType=FromGeometry  MarkerShape=Sphere  MarkerSize=10  GraphicVisPropType=SimpleVisualProperties  GraphicDiffuseColor=[0.6 0.0 0.2]  GraphicSpecularColor=[0.5 0.5 0.5 1.0]  GraphicAmbientColor=[0.15 0.15 0.15 1.0]  GraphicEmissiveColor=[0.0 0.0 0.0 1.0]  GraphicShininess=75  GraphicOpacity=1.0
  Integrator : Integrator
  Propeller4 : sm_lib/Body Elements/File Solid  ExtGeomFileName=E:\tosort\aerial\my new version\propeller.STEP  UnitType=FromFile  ExtGeomFileUnits=m  StepReaderType=HEX  ExportConvexHullGeometry=off  InertiaType=Custom  Mass=0.0249468  MassUnits=kg  CenterOfMass="[0  0.00566766 0]"  CenterOfMassUnits=m  MomentsOfInertia=[0.000160013, 0.000160582, 8.20018e-07]  MomentsOfInertiaUnits=kg*m^2  ProductsOfInertia=[0 0 0]  ProductsOfInertiaUnits=kg*m^2  BasedOnType=Density  Density=1  DensityUnits=g/cm^3  DoExposeReferenceFrame=off  SerializedFrames=<Frames><Frame><Id>Frame1</Id><Value><Name>F1</Name><Origin><Source>GeometricFeature</Source><FeatureName>circular curve 14</FeatureName></Origin><PrimaryAxis><DefinedDirection>+Z</DefinedDirection><Source>ReferenceFrame</Source><SourceDirection>+Y</SourceDirection><FeatureName></FeatureName></PrimaryAxis><SecondaryAxis><DefinedDirection>+X</DefinedDirection><Source>ReferenceFrame</Source><SourceDirection>+X</SourceDirection><FeatureName></FeatureName></SecondaryAxis></Value></Frame></Frames>  GraphicType=FromGeometry  MarkerShape=Sphere  MarkerSize=10  GraphicVisPropType=AdvancedVisualProperties  GraphicDiffuseColor=[0.05 0.05 0.05]  GraphicSpecularColor=[0.5 0.5 0.5 1.0]  GraphicAmbientColor=[0.15 0.15 0.15 1.0]  GraphicEmissiveColor=[0.0 0.0 0.0 1.0]  GraphicShininess=40  GraphicOpacity=1.0
  Revolute Joint : sm_lib/Joints/Revolute Joint  JointMode=Normal  SenseConstraintForce=off  SenseConstraintForceX=off  SenseConstraintForceY=off  SenseConstraintForceZ=off  SenseConstraintTorque=off  SenseConstraintTorqueX=off  SenseConstraintTorqueY=off  SenseConstraintTorqueZ=off  SenseTotalForce=off  SenseTotalForceX=off  SenseTotalForceY=off  SenseTotalForceZ=off  SenseTotalTorque=off  SenseTotalTorqueX=off  SenseTotalTorqueY=off  SenseTotalTorqueZ=off  CompositeWrenchDir=FollowerOnBase  CompositeWrenchFrame=BaseFrame  EquilibriumPosition=0  EquilibriumPositionUnits=deg  SpringStiffness=0  SpringStiffnessUnits=N*m/rad  DampingCoefficient=1e-5  DampingCoefficientUnits=N*m/(rad/s)  TorqueActuationMode=ComputedTorque  MotionActuationMode=InputMotion  SensePosition=off  SenseVelocity=off  SenseAcceleration=off  SenseTorqueForce=off  SenseLowerLimitTorqueForce=off  SenseUpperLimitTorqueForce=off  LowerLimitSpecify=off  LowerLimitBound=-90  LowerLimitBoundUnits=deg  LowerLimitStiffness=1e4  LowerLimitStiffnessUnits=N*m/deg  LowerLimitDamping=10  LowerLimitDampingUnits=N*m/(deg/s)  LowerLimitTransitionRegionWidth=0.1  LowerLimitTransitionRegionWidthUnits=deg  UpperLimitSpecify=off  UpperLimitBound=90  UpperLimitBoundUnits=deg  UpperLimitStiffness=1e4  UpperLimitStiffnessUnits=N*m/deg  UpperLimitDamping=10  UpperLimitDampingUnits=N*m/(deg/s)  UpperLimitTransitionRegionWidth=0.1  UpperLimitTransitionRegionWidthUnits=deg  PositionTargetSpecify=off  PositionTargetPriority=High  PositionTargetValue=0  PositionTargetValueUnits=deg  VelocityTargetSpecify=off  VelocityTargetPriority=High  VelocityTargetValue=0  VelocityTargetValueUnits=deg/s
  Simulink-PS Converter1 : nesl_utility/Simulink-PS Converter  PhysicalDomain=network_engine_domain  SubClassName=ps_input  LeftPortType=input  RightPortType=output  PseudoPeriodic=off  Frequencies=[]  NoiseDistribution=none  NoiseParameters=[]  Unit=rad  AffineConversion=off  FilteringAndDerivatives=filter  SimscapeFilterOrder=2  InputFilterTimeConstant=0.001  UdotUserProvided=0
      settings: SourceProductBaseCode=PW,SS
  P4 : PMIOPort  Side=Left
  wires:
  Integrator/1 -> Simulink-PS Converter1/1
  Input/1 -> Integrator/1
  connections:
  Simulink-PS Converter1/RConn1 -- Revolute Joint/LConn2
  Housing/LConn1 -- Revolute Joint/RConn1
  P4/RConn1 -- Revolute Joint/LConn1
  Housing/RConn1 -- Propeller4/LConn1
